simulink model "sim_aut_dual_scen"  (R2025b)
settings: Solver=ode45  StartTime=0.0  StopTime=Tfin  FixedStep=1e-3  MaxStep=1e-2  MinStep=1e-3  RelTol=5e-3
values from neighbouring files (symbols this model uses):
  bp = [-1.25 -1.19897959184 -1.14795918367 -1.09693877551 -1.04591836735 -0.994897959184 -0.94387755102 -0.892857142857 -0.841836734694 -0.790816326531 -0.739795918367 -0.688775510204 ... (50 elements, 1x50)]    [tire_model.mat]
  C1 = 2.7e4    (= 27000)    [main.m]    (also in model.m)
  C2 = 2e4    (= 20000)    [main.m]    (also in model.m)
  Jz = 4000    [main.m]    (also in model.m)
  K = nmpc_design_st2(par,2)    [main.m]
  l1 = 1.2    [main.m]    (also in model.m)
  l2 = 1.6    [main.m]    (also in model.m)
  m = 1575    [main.m]    (also in model.m)
  Np = round(vx_ref*K.Tp/mean(ds))    [main.m]
  pacf = [2550.90487699 2674.70463742 2810.77279096 2960.97362657 3127.55760929 3313.26346728 3521.4532226 3756.29269015 4022.99538347 4328.15571957 4680.20907939 5090.07319782 ... (50 elements, 1x50)]    [tire_model.mat]
  pacr = [2550.90487699 2674.70463742 2810.77279096 2960.97362657 3127.55760929 3313.26346728 3521.4532226 3756.29269015 4022.99538347 4328.15571957 4680.20907939 5090.07319782 ... (50 elements, 1x50)]    [tire_model.mat]
  psi = x(3)    [model.m]
  psir = [atan2(diff(Yr),diff(Xr));0]    [main.m]
  refPoses = [Xr,Yr,psir]    [main.m]
  Ts = 0.05    [main.m]
  ze0 = [X0;Y0;psi0;vx0;vy0;wpsi0]    [main.m]
undefined symbols (not defined in the file or in its folder): aMode, plot_ref, x_o
libraries: autolibsharedcommon x11, autolibshared x5, autolibpowerinfoutils x2, autolibutils x2, sharedtransform x2, simulink x1, drivingscenarioandsensors x1
(part 1 of 4)
settings Model: PacingRate=0.750000  Creator=The MathWorks, Inc.  LastModifiedBy=denni
settings SolverCC: ZeroCrossAlgorithm=Adaptive  AlgebraicLoopSolver=TrustRegion  DecoupledContinuousIntegration=on  MinimalZcImpactIntegration=on
settings DataIOCC: SaveOutput=off  DSMLogging=off  SaveTime=off  ReturnWorkspaceOutputs=off
settings DebuggingCC: UnconnectedInputMsg=warning  UnconnectedOutputMsg=warning  UnconnectedLineMsg=warning  ArithmeticOperatorsInVariantConditions=warning
settings ModelReferenceCC: EnableRefExpFcnMdlSchedulingChecks=on  PropagateSignalLabelsOutOfModel=off
settings SFSimCC: SimUseLocalCustomCode=off  CustomCodeUndefinedFunction=UseInterfaceOnly
settings RTWCC: RTWUseLocalCustomCode=off  GPUComputeCapability=3.5  DLArmComputeVersion=19.05

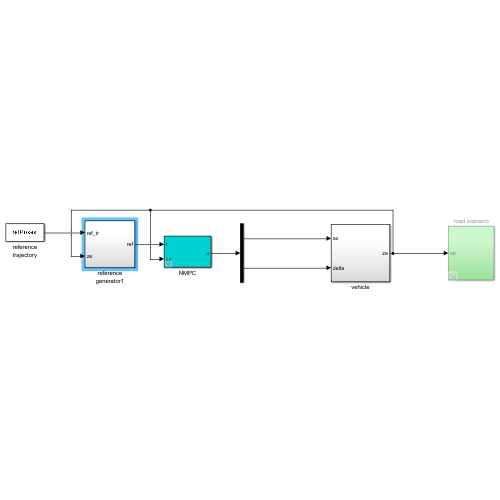
[thumbnail: Simulink's stored preview of the top-level diagram]
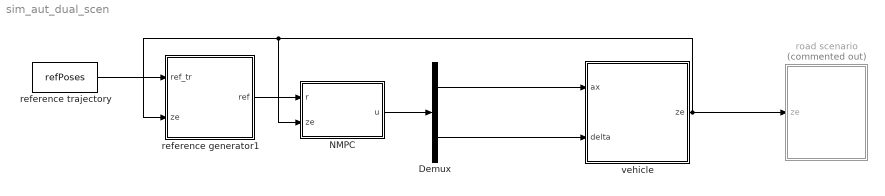
== system sim_aut_dual_scen ==
  Demux : Demux  Outputs=2
  NMPC : Subsystem  mask{K=K}
      mask prompts: K "NMPC structure"
  reference generator1 : Subsystem
  reference trajectory : Constant  Value=refPoses
  road scenario : Subsystem  Commented=on
      settings: PortSchema="{\"entries\":[{\"content\":{\"sides\":[{\"content\":{},\"type\":\"ConnectorPlacement.EquallySpacedRectSide\",\"uuid\":\"f0897155-b1ca-4bdd-a38e-3494662c4a0b\"},{\"content\":{\"connectorIds\":[\"In1\"],\"side\":\"RIGHT\"},\"type\":\"ConnectorPlacement.EquallySpacedRectSide\",\"uuid\":\"ba8f9432-9c07-44a3-8769-5c417be23bfd\"},{\"content\":{\"side\":\"TOP\"},\"type\":\"ConnectorPlacement.EquallySpacedRectSide\",\"uuid\":\"74ba7e9d-4aff-4913-b94c-95c9a4f4fd7f\"}]},\"type\":\"ConnectorPlacement.EquallySpacedConnector\",\"uuid\":\"ef070011-996a-4f52-a3ae-9ceda936acba\"}],\"packageUris\":[\"http://schema.mathworks.com/mf0/Connector/R2020b\"],\"version\":\"1.0\"}"
  vehicle : Subsystem
  wires:
  vehicle/1(ze) -> reference generator1/2(ze), NMPC/2(ze), road scenario/1(ze)
  reference trajectory/1 -> reference generator1/1(ref_tr)
  NMPC/1(u) -> Demux/1
  reference generator1/1(ref) -> NMPC/1(r)
  Demux/2 -> vehicle/2(delta)
  Demux/1 -> vehicle/1(ax)

== system sim_aut_dual_scen/NMPC ==
  r : Inport
  ze : Inport  Port=2
  Clock : Clock
  Mux2 : Mux
  Rate Transition{1..4} (4 alike) : RateTransition  OutPortSampleTime=K.Ts
  Selector1 : Selector  InputPortWidth=K.nc  IndexOptions=Index vector (dialog)  Indices=1:K.nu  OutputSizes=1
  Unit Delay : UnitDelay  InitialCondition=zeros(K.nc,1)  SampleTime=K.Ts  HasFrameUpgradeWarning=on
  nmpc : MATLABFcn  MATLABFcn=nmpc_st2(K,u(1:K.nx),u(K.nx+1:K.nx+K.nc),u(K.nx+K.nc+1:end-1),u(end))  OutputDimensions=K.nc
  u : Outport
  wires:
  ze/1 -> Rate Transition2/1
  Unit Delay/1 -> Mux2/2, Rate Transition1/1
  Mux2/1 -> nmpc/1
  r/1 -> Rate Transition3/1
  Rate Transition2/1 -> Mux2/1
  Rate Transition1/1 -> Selector1/1
  Rate Transition3/1 -> Mux2/3
  nmpc/1 -> Unit Delay/1
  Selector1/1 -> u/1
  Clock/1 -> Rate Transition4/1
  Rate Transition4/1 -> Mux2/4

== system sim_aut_dual_scen/reference generator1 ==
  ref_tr : Inport
  ze : Inport  Port=2
  Constant : Constant  Value=Np
  Demux : Demux
  Gain : Gain  Gain=[0 0 0 3.6 0 0]  Multiplication=Matrix(K*u)
  Gain1 : Gain  Gain=-1
  MATLAB Function1 : MATLAB Function  TreatAsAtomicUnit=on
  Mux : Mux  Inputs=2
  Mux1 : Mux  Inputs=2
  Scope3 : Scope  NumInputPorts=3
      settings: ActiveDisplayYMinimum=-0.12618507931424761  ActiveDisplayYMaximum=0.15446039878025969  DataLoggingVariableName=ScopeData2
  Subsystem : Subsystem
  To Workspace1 : ToWorkspace  VariableName=errors  SaveFormat=Timeseries  SampleTime=-1
  To Workspace2 : ToWorkspace  VariableName=e_ct  SaveFormat=Timeseries  SampleTime=-1
  ref : Outport
  wires:
  ref_tr/1 -> MATLAB Function1/2(ref_tr)
  ze/1 -> Gain/1, Subsystem/3(ze), MATLAB Function1/3(ze)
  MATLAB Function1/2(ref_pose) -> Subsystem/2(ref_pose)
  Subsystem/1(ee) -> Demux/1
  Subsystem/2(e_ct) -> Mux1/1, To Workspace2/1
  Mux/1 -> To Workspace1/1
  Gain/1 -> Scope3/3
  MATLAB Function1/1(ref) -> Subsystem/1(ref XY), ref/1
  Constant/1 -> MATLAB Function1/1(Np)
  Demux/1 -> Gain1/1, Mux/1
  Demux/2 -> Scope3/2, Mux/2
  Mux1/1 -> Scope3/1
  Gain1/1 -> Mux1/2

== system sim_aut_dual_scen/road scenario ==
  ze : Inport
  MATLAB Function1 : MATLAB Function  TreatAsAtomicUnit=on
  Scenario Reader : drivingscenarioandsensors/Scenario Reader  ScenarioSource=From workspace  ScenarioFileName=EgoVehicleGoesStraight.mat  ScenarioVariableName=scenario  OutputCoordinateSystem=Vehicle coordinates  EgoVehicleSource=Input port  EgoVehicleActorID=1  OrientVehiclesOnRoad=on  OutputEgoVehiclePose=on  OutputEgoVehicleState=on  SampleTime=0.1  LaneBoundaryOutput=All lane boundaries  LaneBoundaryDistance=0:0.5:9.5  LaneBoundaryLocation=Center of lane markings  BusNameSource=Auto  BusName=ActorPose  BusNumActorsSource=Scenario  BusNumActors=3  BusName2Source=Auto  BusName2=BusLaneBoundaries  BusNumLaneBoundariesSource=Scenario  BusNumLaneBoundaries=10  BusName3Source=Auto  BusName3=BusEgoActor  BusName4Source=Auto  BusName4=BusEgoState  ShowCoordinateLabels=on  SimulateUsing=Interpreted execution
  Terminator : Terminator
  Terminator1 : Terminator
  wires:
  MATLAB Function1/1(egoPose) -> Scenario Reader/1
  Scenario Reader/1 -> Terminator/1
  Scenario Reader/2 -> Terminator1/1
  ze/1 -> MATLAB Function1/1(ze)

== system sim_aut_dual_scen/vehicle ==
  ax : Inport
  delta : Inport  Port=2
  Actuator : TransferFcn  Denominator=[0.1 1]
  Rate Transition3 : RateTransition  InitialCondition=ze0  OutPortSampleTime=Ts
  Saturation : Saturate  UpperLimit=0.4  LowerLimit=-0.4
  Saturation1 : Saturate  UpperLimit=3  LowerLimit=-10
  Scope1 : Scope  NumInputPorts=2
      settings: ActiveDisplayYMinimum=-11.625  ActiveDisplayYMaximum=4.625
  Scope2 : Scope  NumInputPorts=2
      settings: ActiveDisplayYMinimum=-0.04592  ActiveDisplayYMaximum=0.31381
  To Workspace : ToWorkspace  VariableName=ze  SaveFormat=Timeseries  SampleTime=-1
  To Workspace1 : ToWorkspace  VariableName=delta  SaveFormat=Timeseries  SampleTime=-1
  To Workspace2 : ToWorkspace  VariableName=ax  SaveFormat=Timeseries  SampleTime=-1
  dual-track : Subsystem
  lower level controller/actuators : TransferFcn  Denominator=[0.5 1]
  ze : Outport  VectorParamsAs1DForOutWhenUnconnected=off
  wires:
  Rate Transition3/1 -> To Workspace/1, ze/1
  delta/1 -> To Workspace1/1, Actuator/1
  Actuator/1 -> Saturation/1
  Saturation/1 -> Scope2/2, dual-track/2(delta)
  lower level controller/actuators/1 -> Saturation1/1
  Saturation1/1 -> Scope2/1, dual-track/1(ax), Scope1/2
  ax/1 -> To Workspace2/1, Scope1/1, lower level controller/actuators/1
  dual-track/1(state) -> Rate Transition3/1

== system sim_aut_dual_scen/reference generator1/Subsystem ==
  ref XY : Inport
  ref_pose : Inport  Port=2
  ze : Inport  Port=3
  Discrete Derivative : simulink/Discrete/Discrete Derivative  gainval=1.0  ICPrevScaledInput=psir(1)/Ts  OutMin=[]  OutMax=[]  OutDataType=fixdt(1, 16)  OutScaling=2^-10  DoSatur=off
  Interpreted MATLAB Function : MATLABFcn  Commented=on  MATLABFcn=plot_ref(u)  OutputDimensions=0
  MATLAB Function2 : MATLAB Function  TreatAsAtomicUnit=on  VariantControl=Choice
  Mux : Mux  Inputs=2
  Rate Transition : RateTransition  Commented=on  OutPortSampleTime=Ts
  Selector2 : Selector  InputPortWidth=3  IndexOptions=Index vector (dialog)  Indices=3  OutputSizes=1
  Terminator : Terminator
  errors : Subsystem
  ee : Outport
  e_ct : Outport  Port=2
  wires:
  MATLAB Function2/1(e_ct) -> e_ct/1
  Discrete Derivative/1 -> errors/2(psi_r_dot)
  ze/1 -> MATLAB Function2/2(ze), errors/3(ze), Mux/1
  Rate Transition/1 -> Interpreted MATLAB Function/1
  errors/1(ee) -> ee/1
  ref XY/1 -> Mux/2
  Mux/1 -> Rate Transition/1
  ref_pose/1 -> MATLAB Function2/1(ref_pose), errors/1(refPoses), Selector2/1
  Selector2/1 -> Discrete Derivative/1
  MATLAB Function2/2(e_h) -> Terminator/1

== system sim_aut_dual_scen/vehicle/dual-track ==
  ax : Inport
  delta : Inport  Port=2
  Bus Selector1 : BusSelector  OutputSignals=InertFrm.Cg.Disp.X,InertFrm.Cg.Disp.Y
  Constant1 : Constant  Value=[0;0]
  Gain1 : Gain  Gain=[1;1]
  Gain2 : Gain  Gain=m*[0.5;0.5]
  Mux2 : Mux  Inputs=6
  Terminator1 : Terminator
  Terminator4 : Terminator
  Vehicle Body 3DOF Dual Track : Subsystem  AncestorBlock=autolibshared/Vehicle Body 3DOF Single Track  mask(Vehicle Body 3DOF Lateral){trackMode=Dual, inputMode=External longitudinal forces, frontSteerMode=on, rearSteerMode=off, windMode=off, muMode=off, extFMode=off, extMMode=off, htchFMode=off, htchMMode=off, extXo=off, extpsio=off, extxdoto=off, extro=off, extYo=off, extTamb=off, extydoto=off, aMode=aMode, NF=2, NR=2, m=m, a=l1, b=l2, h=0.35, dh=1, hh=0.2, X_o=ze0(1), xdot_o=ze0(4), CalphaMode=off, sigmaMode=on, d=0, hl=0, w=[1.4,1.4], Cy_f=C1, Cy_r=C2, sigma_f=.1, sigma_r=.1, alpha_f_brk=[-.1 .1], Cy_f_data=[-9e3 9e3], alpha_r_brk=[-.1 .1], Cy_r_data=[-9e3 9e3], Y_o=ze0(2), ydot_o=ze0(5), Izz=Jz, psi_o=ze0(3), r_o=ze0(6), Af=2, Cd=.3, Cl=.1, Cpm=.1, beta_w=[0 0.01:0.01:0.3], Cs=[0 0.01:0.01:0.3], Cym=[0 1e-6:0.01:0.3], Pabs=101325, Tair=273, g=9.81, mu=1, xdot_tol=.01, Fznom=5000, Fxtire_sat=1e6, Fytire_sat=1e6, longOff=0, latOff=0, vertOff=0, wrapAng=off}
      mask prompts: trackMode "autoblks_shared:autoblkVehBody3DofLat:blkPrm_trackMode"; inputMode "autoblks_shared:autoblkVehBody3DofLat:blkPrm_inputMode"; frontSteerMode "autoblks_shared:autoblkVehBody3DofLat:blkPrm_frontSteerMode"; rearSteerMode "autoblks_shared:autoblkVehBody3DofLat:blkPrm_rearSteerMode"; windMode "autoblks_shared:autoblkVehBody3DofLat:blkPrm_windMode"; muMode "autoblks_shared:autoblkVehBody3DofLat:blkPrm_muMode"; extFMode "autoblks_shared:autoblkVehBody3DofLat:blkPrm_extFMode"; extMMode "autoblks_shared:autoblkVehBody3DofLat:blkPrm_extMMode"; htchFMode "autoblks_shared:autoblkVehBody3DofLat:blkPrm_htchFMode"; htchMMode "autoblks_shared:autoblkVehBody3DofLat:blkPrm_htchMMode"; extXo "autoblks_shared:autoblkVehBody3DofLat:blkPrm_extXo"; extpsio "autoblks_shared:autoblkVehBody3DofLat:blkPrm_extpsio"; extxdoto "autoblks_shared:autoblkVehBody3DofLat:blkPrm_extxdoto"; extro "autoblks_shared:autoblkVehBody3DofLat:blkPrm_extro"; extYo "autoblks_shared:autoblkVehBody3DofLat:blkPrm_extYo"; extTamb "autoblks_shared:autoblkVehBody3DofLat:blkPrm_extTamb"; extydoto "autoblks_shared:autoblkVehBody3DofLat:blkPrm_extydoto"; NF "autoblks_shared:autoblkVehBody3DofLat:blkPrm_NF"; NR "autoblks_shared:autoblkVehBody3DofLat:blkPrm_NR"; m "autoblks_shared:autoblkVehBody3DofLat:blkPrm_m"; a "autoblks_shared:autoblkVehBody3DofLat:blkPrm_a"; b "autoblks_shared:autoblkVehBody3DofLat:blkPrm_b"; h "autoblks_shared:autoblkVehBody3DofLat:blkPrm_h"; dh "autoblks_shared:autoblkVehBody3DofLat:blkPrm_dh"; hh "autoblks_shared:autoblkVehBody3DofLat:blkPrm_hh"; X_o "autoblks_shared:autoblkVehBody3DofLat:blkPrm_X_o"; xdot_o "autoblks_shared:autoblkVehBody3DofLat:blkPrm_xdot_o"; CalphaMode "autoblks_shared:autoblkVehBody3DofLat:blkPrm_CalphaMode"; sigmaMode "autoblks_shared:autoblkVehBody3DofLat:blkPrm_sigmaMode"; d "autoblks_shared:autoblkVehBody3DofLat:blkPrm_d"; hl "autoblks_shared:autoblkVehBody3DofLat:blkPrm_hl"; w "autoblks_shared:autoblkVehBody3DofLat:blkPrm_w"; Cy_f "autoblks_shared:autoblkVehBody3DofLat:blkPrm_Cy_f"; Cy_r "autoblks_shared:autoblkVehBody3DofLat:blkPrm_Cy_r"; sigma_f "autoblks_shared:autoblkVehBody3DofLat:blkPrm_sigma_f"; sigma_r "autoblks_shared:autoblkVehBody3DofLat:blkPrm_sigma_r"; alpha_f_brk "autoblks_shared:autoblkVehBody3DofLat:blkPrm_alpha_f_brk"; Cy_f_data "autoblks_shared:autoblkVehBody3DofLat:blkPrm_Cy_f_data"; alpha_r_brk "autoblks_shared:autoblkVehBody3DofLat:blkPrm_alpha_r_brk"; Cy_r_data "autoblks_shared:autoblkVehBody3DofLat:blkPrm_Cy_r_data"; Y_o "autoblks_shared:autoblkVehBody3DofLat:blkPrm_Y_o"; ydot_o "autoblks_shared:autoblkVehBody3DofLat:blkPrm_ydot_o"; Izz "autoblks_shared:autoblkVehBody3DofLat:blkPrm_Izz"; psi_o "autoblks_shared:autoblkVehBody3DofLat:blkPrm_psi_o"; r_o "autoblks_shared:autoblkVehBody3DofLat:blkPrm_r_o"; Af "autoblks_shared:autoblkVehBody3DofLat:blkPrm_Af"; Cd "autoblks_shared:autoblkVehBody3DofLat:blkPrm_Cd"; Cl "autoblks_shared:autoblkVehBody3DofLat:blkPrm_Cl"; Cpm "autoblks_shared:autoblkVehBody3DofLat:blkPrm_Cpm"; beta_w "autoblks_shared:autoblkVehBody3DofLat:blkPrm_beta_w"; Cs "autoblks_shared:autoblkVehBody3DofLat:blkPrm_Cs"; Cym "autoblks_shared:autoblkVehBody3DofLat:blkPrm_Cym"; Pabs "autoblks_shared:autoblkVehBody3DofLat:blkPrm_Pabs"; Tair "autoblks_shared:autoblkVehBody3DofLat:blkPrm_Tair"; g "autoblks_shared:autoblkVehBody3DofLat:blkPrm_g"; mu "autoblks_shared:autoblkVehBody3DofLat:blkPrm_mu"; xdot_tol "autoblks_shared:autoblkVehBody3DofLat:blkPrm_xdot_tol"; Fznom "autoblks_shared:autoblkVehBody3DofLat:blkPrm_Fznom"; Fxtire_sat "autoblks_shared:autoblkVehBody3DofLat:blkPrm_Fxtire_sat"; Fytire_sat "autoblks_shared:autoblkVehBody3DofLat:blkPrm_Fytire_sat"; longOff "autoblks_shared:autoblkVehBody3DofLat:blkPrm_longOff"; latOff "autoblks_shared:autoblkVehBody3DofLat:blkPrm_latOff"; vertOff "autoblks_shared:autoblkVehBody3DofLat:blkPrm_vertOff"; wrapAng "autoblks_shared:autoblkVehBody3DofLat:blkPrm_wrapAng"
      mask help: autoblks_shared:autoblkVehBody3DofLat:blkDesc
      mask init:
      | [~]=autosharedicon('vehdynliblat3dof',gcb,0);
      mask Help: eval('autosharedhelp(''vb3doflat'')');
      mask TypeOptions trackMode: autoblks_shared:autoblkVehBody3DofLat:blkCmb_trackMode_c1 | autoblks_shared:autoblkVehBody3DofLat:blkCmb_trackMode_c2
      mask Callback trackMode: [~]=autosharedicon('vehdynliblat3dof',gcb,5);
      mask TypeOptions inputMode: autoblks_shared:autoblkVehBody3DofLat:blkCmb_inputMode_c1 | autoblks_shared:autoblkVehBody3DofLat:blkCmb_inputMode_c2 | autoblks_shared:autoblkVehBody3DofLat:blkCmb_inputMode_c3
      mask Callback inputMode: [~]=autosharedicon('vehdynliblat3dof',gcb,1);
      mask Callback muMode: [~]=autosharedicon('vehdynliblat3dof',gcb,2);
      mask Callback extXo: [~]=autosharedicon('vehdynliblat3dof',gcb,7);
      mask Callback extpsio: [~]=autosharedicon('vehdynliblat3dof',gcb,7);
      mask Callback extxdoto: [~]=autosharedicon('vehdynliblat3dof',gcb,7);
      mask Callback extro: [~]=autosharedicon('vehdynliblat3dof',gcb,7);
      mask Callback extYo: [~]=autosharedicon('vehdynliblat3dof',gcb,7);
      mask Callback extTamb: [~]=autosharedicon('vehdynliblat3dof',gcb,6);
      mask Callback extydoto: [~]=autosharedicon('vehdynliblat3dof',gcb,7);
      mask Callback CalphaMode: [~]=autosharedicon('vehdynliblat3dof',gcb,3);
      mask Callback sigmaMode: [~]=autosharedicon('vehdynliblat3dof',gcb,4);
      mask DialogControl blockConfig Prompt: autoblks_shared:autoblkVehBody3DofLat:blkDlg_blockConfig
      mask DialogControl trackMode Prompt: Vehicle track:
      mask DialogControl inputMode Prompt: Axle forces:
      mask DialogControl extModePanel Prompt: autoblks_shared:autoblkVehBody3DofLat:blkDlg_extModePanel
      mask DialogControl frontSteerMode Prompt: Front wheel steering
      mask DialogControl rearSteerMode Prompt: Rear wheel steering
      mask DialogControl windMode Prompt: External wind
      mask DialogControl muMode Prompt: External friction
      mask DialogControl extFMode Prompt: External forces
      mask DialogControl extMMode Prompt: External moments
      mask DialogControl htchFMode Prompt: Hitch forces
      mask DialogControl htchMMode Prompt: Hitch moments
      mask DialogControl extXo Prompt: Initial longitudinal position
      mask DialogControl extpsio Prompt: Initial yaw angle
      mask DialogControl extxdoto Prompt: Initial longitudinal velocity
      mask DialogControl extro Prompt: Initial yaw rate
      mask DialogControl extYo Prompt: Initial lateral position
      mask DialogControl extTamb Prompt: Air temperature
      mask DialogControl extydoto Prompt: Initial lateral velocity
      mask DialogControl ParameterGroupVar Prompt: autoblks_shared:autoblkVehBody3DofLat:blkDlg_ParameterGroupVar
      mask DialogControl LongPanel Prompt: autoblks_shared:autoblkVehBody3DofLat:blkDlg_LongPanel
      mask DialogControl NF Prompt: Number of wheels on front axle, NF [-]:
      mask DialogControl NR Prompt: Number of wheels on rear axle, NR [-]:
      mask DialogControl m Prompt: Vehicle mass, m [kg]:
      mask DialogControl a Prompt: Longitudinal distance from center of mass to front axle, a [m]:
      mask DialogControl b Prompt: Longitudinal distance from center of mass to rear axle, b [m]:
      mask DialogControl h Prompt: Vertical distance from center of mass to axle plane, h [m]:
      mask DialogControl dh Prompt: Longitudinal distance from center of mass to hitch, dh [m]:
      mask DialogControl hh Prompt: Vertical distance from hitch to axle plane, hh [m]:
      mask DialogControl X_o Prompt: Initial inertial frame longitudinal position, X_o [m]:
      mask DialogControl xdot_o Prompt: Initial longitudinal velocity, xdot_o [m/s]:
      mask DialogControl LatPanel Prompt: autoblks_shared:autoblkVehBody3DofLat:blkDlg_LatPanel
      mask DialogControl CalphaMode Prompt: Mapped corner stiffness:
      mask DialogControl sigmaMode Prompt: Include relaxation length dynamics:
      mask DialogControl d Prompt: Lateral distance from geometric centerline to center of mass, d [m]:
      mask DialogControl hl Prompt: Lateral distance from geometric centerline to hitch, hl [m]:
      mask DialogControl w Prompt: Track width, w [m]:
      mask DialogControl Cy_f Prompt: Front tire corner stiffness, Cy_f [N/rad]:
      mask DialogControl Cy_r Prompt: Rear tire corner stiffness, Cy_r [N/rad]:
      mask DialogControl sigma_f Prompt: Front tire(s) relaxation length, sigma_f [m]:
      mask DialogControl sigma_r Prompt: Rear tire(s) relaxation length, sigma_r [m]:
      mask DialogControl alpha_f_brk Prompt: Front axle slip angle breakpoints, alpha_f_brk [rad]:
      mask DialogControl Cy_f_data Prompt: Front axle corner data, Cy_f_data [N/rad]:
      mask DialogControl alpha_r_brk Prompt: Rear axle slip angle breakpoints, alpha_r_brk [rad]:
      mask DialogControl Cy_r_data Prompt: Rear axle corner data, Cy_r_data [N/rad]:
      mask DialogControl Y_o Prompt: Initial inertial frame lateral displacement, Y_o [m]:
      mask DialogControl ydot_o Prompt: Initial lateral velocity, ydot_o [m/s]:
      mask DialogControl YawPanel Prompt: autoblks_shared:autoblkVehBody3DofLat:blkDlg_YawPanel
      mask DialogControl Izz Prompt: Yaw polar inertia, Izz [kg*m^2]:
      mask DialogControl psi_o Prompt: Initial yaw angle, psi_o [rad]:
      mask DialogControl r_o Prompt: Initial yaw rate, r_o [rad/s]:
      mask DialogControl AeroParams Prompt: autoblks_shared:autoblkVehBody3DofLat:blkDlg_AeroParams
      mask DialogControl Af Prompt: Longitudinal drag area, Af [m^2]:
      mask DialogControl Cd Prompt: Longitudinal drag coefficient, Cd [-]:
      mask DialogControl Cl Prompt: Longitudinal lift coefficient, Cl [-]:
      mask DialogControl Cpm Prompt: Longitudinal drag pitch moment, Cpm [-]:
      mask DialogControl beta_w Prompt: Relative wind angle vector, beta_w [rad]:
      mask DialogControl Cs Prompt: Side force coefficient vector, Cs [-]:
      mask DialogControl Cym Prompt: Yaw moment coefficient vector, Cym [-]:
      mask DialogControl EnviroPanel Prompt: autoblks_shared:autoblkVehBody3DofLat:blkDlg_EnviroPanel
      mask DialogControl Pabs Prompt: Absolute pressure, Pabs [Pa]:
      mask DialogControl Tair Prompt: Air temperature, Tair [K]:
      mask DialogControl g Prompt: Gravitational acceleration, g [m/s^2]:
      mask DialogControl mu Prompt: Nominal friction scaling factor, mu [-]:
      mask DialogControl SimPanel Prompt: autoblks_shared:autoblkVehBody3DofLat:blkDlg_SimPanel
      mask DialogControl xdot_tol Prompt: Longitudinal velocity tolerance, xdot_tol [m/s]:
      mask DialogControl Fznom Prompt: Nominal normal force, Fznom [N]:
      mask DialogControl Fxtire_sat Prompt: Longitudinal force limit, Fxtire_sat [N]:
      mask DialogControl Fytire_sat Prompt: Lateral force limit, Fytire_sat [N]:
      mask DialogControl longOff Prompt: Geometric longitudinal offset from axle plane, longOff [m]:
      mask DialogControl latOff Prompt: Geometric lateral offset from center plane, latOff [m]:
      mask DialogControl vertOff Prompt: Geometric vertical offset from axle plane, vertOff [m]:
      mask DialogControl wrapAng Prompt: Wrap Euler angles, wrapAng
      mask Display:
      | try
      |     IconInfo = autosharedicon('vehdynliblat3dof',gcb,8);
      | 
      |     image(IconInfo.image, IconInfo.position);
      | 
      |     for i = 1:numel(IconInfo.lconn)
      |         port_label('lconn', i, IconInfo.lconn{i})
      |     end
      | 
      |     for j = 1:numel(IconInfo.rconn)
      |         port_label('rconn', j, IconInfo.rconn{j})
      |     end
      | 
      |     for k = 1:numel(IconInfo.input)
      |         port_label('input', k, IconInfo.input{k})
      |     end
      | 
      |     for m = 1:numel(IconInfo.output)
      |         port_label('output', m, IconInfo.output{m})
      |     end
      | catch
      |     fprintf('Vehicle Body \n 3DOF Lateral')
      | end
  state : Outport
  wires:
  delta/1 -> Gain1/1
  Vehicle Body 3DOF Dual Track/4(psi) -> Mux2/3
  Vehicle Body 3DOF Dual Track/6(FzF) -> Terminator1/1
  Vehicle Body 3DOF Dual Track/5(r) -> Mux2/6
  Vehicle Body 3DOF Dual Track/7(FzR) -> Terminator4/1
  Gain1/1 -> Vehicle Body 3DOF Dual Track/1(WhlAngF)
  Bus Selector1/1 -> Mux2/1  "<X>"
  Vehicle Body 3DOF Dual Track/1(Info) -> Bus Selector1/1
  Constant1/1 -> Vehicle Body 3DOF Dual Track/3(FwR)
  Vehicle Body 3DOF Dual Track/3(ydot) -> Mux2/5
  Vehicle Body 3DOF Dual Track/2(xdot) -> Mux2/4
  ax/1 -> Gain2/1
  Bus Selector1/2 -> Mux2/2  "<Y>"
  Mux2/1 -> state/1  "state"
  Gain2/1 -> Vehicle Body 3DOF Dual Track/2(FwF)

== system sim_aut_dual_scen/reference generator1/Subsystem/errors ==
  refPoses : Inport
  psi_r_dot : Inport  Port=2
  ze : Inport  Port=3
  Integrator : Integrator
  MATLAB Function : MATLAB Function  TreatAsAtomicUnit=on
  Mux : Mux
  ee : Outport
  wires:
  Integrator/1 -> Mux/1
  MATLAB Function/2(e_psi) -> Mux/2
  MATLAB Function/3(e_psi_dot) -> Mux/4
  MATLAB Function/1(e_y_dot) -> Mux/3, Integrator/1
  Mux/1 -> ee/1
  psi_r_dot/1 -> MATLAB Function/2(psi_r_dot)
  ze/1 -> MATLAB Function/3(ze)
  refPoses/1 -> MATLAB Function/1(ref)

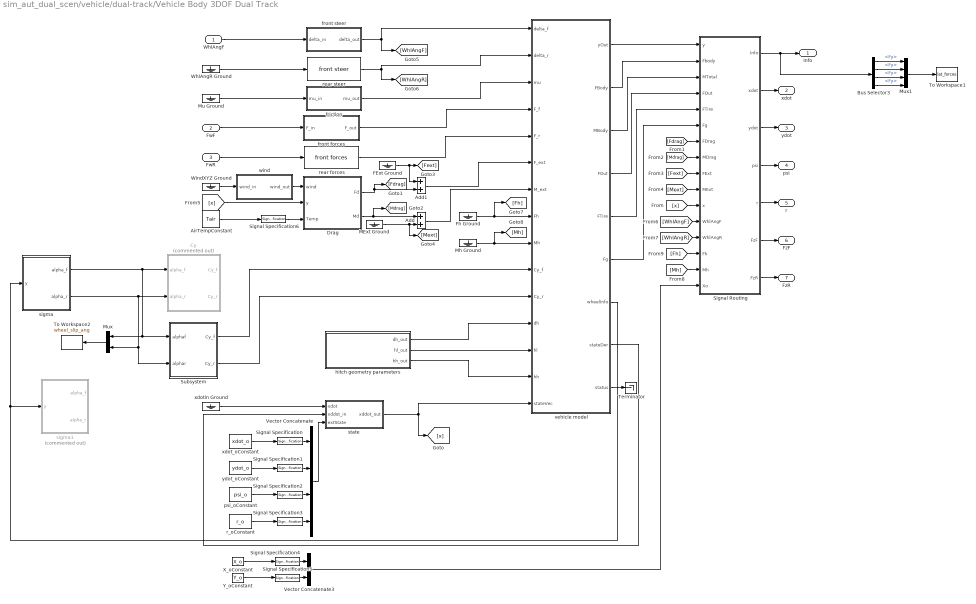
== system sim_aut_dual_scen/vehicle/dual-track/Vehicle Body 3DOF Dual Track ==
  WhlAngF : Inport
  FwF : Inport  Port=2
  FwR : Inport  Port=3
  Add : Sum
  Add1 : Sum
  AirTempConstant : Constant  Value=Tair
  Bus Selector3 : BusSelector  OutputSignals=BdyFrm.Forces.Tires.FrntTires.Lft.Fy,BdyFrm.Forces.Tires.FrntTires.Rght.Fy,BdyFrm.Forces.Tires.RearTires.Lft.Fy,BdyFrm.Forces.Tires.RearTires.Rght.Fy
  Cy : Subsystem  Commented=on  Variant=on  VariantControlMode=label  LabelModeActiveChoice=2
  Drag : Subsystem
  FExt Ground : Ground
  Fh Ground : Ground
  MExt Ground : Ground
  Mh Ground : Ground
  Mu Ground : Ground
  Mux : Mux  Inputs=2
  Mux1 : Mux
  Signal Routing : Subsystem  Variant=on  VariantControlMode=label  LabelModeActiveChoice=1
  Signal Specification : SignalSpecification  Unit=m/s
  Signal Specification1 : SignalSpecification  Unit=m/s
  Signal Specification2 : SignalSpecification  Unit=rad
  Signal Specification3 : SignalSpecification  Unit=rad/s
  Signal Specification4 : SignalSpecification  Unit=m
  Signal Specification5 : SignalSpecification  Unit=m
  Signal Specification6 : SignalSpecification  Unit=K
  Subsystem : Subsystem
  Terminator : Terminator
  To Workspace1 : ToWorkspace  VariableName=lat_forces  SaveFormat=Timeseries  SampleTime=Ts
  To Workspace2 : ToWorkspace  VariableName=wheel_slip_ang  SaveFormat=Timeseries  SampleTime=Ts
  Vector Concatenate : Concatenate  NumInputs=4
  Vector Concatenate3 : Concatenate
  WhlAngR Ground : Ground
  WindXYZ Ground : Ground
  X_oConstant : Constant  Value=X_o
  Y_oConstant : Constant  Value=Y_o
  friction : Subsystem  Variant=on  VariantControlMode=label  LabelModeActiveChoice=2
  front forces : Subsystem  Variant=on  VariantControlMode=label  LabelModeActiveChoice=4
  front steer : Subsystem  Variant=on  VariantControlMode=label  LabelModeActiveChoice=3
  hitch geometry parameters : Subsystem  Variant=on  VariantControlMode=label  LabelModeActiveChoice=3
  psi_oConstant : Constant  Value=psi_o
  r_oConstant : Constant  Value=r_o
  rear forces : autolibshared/Vehicle Body 3DOF Single Track/front forces  SystemSampleTime=-1  LabelModeActiveChoice=4  VariantActivationTime=update diagram  EmptyChoice=off  PassThrough=off  PassThroughVariantControl=(default)  EmptyChoiceVariantControl=(default)  AllowFlexibleInterface=on  Latency=0  AutoFrameSizeCalculation=off
  rear steer : autolibshared/Vehicle Body 3DOF Single Track/front steer  SystemSampleTime=-1  LabelModeActiveChoice=2  VariantActivationTime=update diagram  EmptyChoice=off  PassThrough=off  PassThroughVariantControl=(default)  EmptyChoiceVariantControl=(default)  AllowFlexibleInterface=on  Latency=0  AutoFrameSizeCalculation=off
  sigma : Subsystem  Variant=on  VariantControlMode=label  LabelModeActiveChoice=3
  sigma1 : Subsystem  Commented=on  Variant=on  VariantControlMode=label  LabelModeActiveChoice=3
  state : Subsystem  Variant=on  VariantControlMode=label  LabelModeActiveChoice=0
  vehicle model : MATLAB Function  TreatAsAtomicUnit=on
  wind : Subsystem  Variant=on  VariantControlMode=label  LabelModeActiveChoice=0
  xdot_oConstant : Constant  Value=xdot_o
  xdotin Ground : Ground
  ydot_oConstant : Constant  Value=ydot_o
  Info : Outport  VectorParamsAs1DForOutWhenUnconnected=off
  xdot : Outport  Port=2  VectorParamsAs1DForOutWhenUnconnected=off
  ydot : Outport  Port=3  VectorParamsAs1DForOutWhenUnconnected=off
  psi : Outport  Port=4  VectorParamsAs1DForOutWhenUnconnected=off
  r : Outport  Port=5  VectorParamsAs1DForOutWhenUnconnected=off
  FzF : Outport  Port=6  VectorParamsAs1DForOutWhenUnconnected=off
  FzR : Outport  Port=7  VectorParamsAs1DForOutWhenUnconnected=off
  wires:
  AirTempConstant/1 -> Signal Specification6/1
  [Fh] -> Signal Routing/14(Fh)
  [Mh] -> Signal Routing/15(Mh)
  hitch geometry parameters/3(hh_out) -> vehicle model/14(hh)
  hitch geometry parameters/2(hl_out) -> vehicle model/13(hl)
  hitch geometry parameters/1(dh_out) -> vehicle model/12(dh)
  Mh Ground/1 -> [Mh], vehicle model/9(Mh)
  Fh Ground/1 -> [Fh], vehicle model/8(Fh)
  FExt Ground/1 -> [Fext], Add1/1
  MExt Ground/1 -> Add/2, [Mext]
  FwR/1 -> rear forces/1
  FwF/1 -> front forces/1(F_in)
  xdotin Ground/1 -> state/1(xdot)
  Signal Specification6/1 -> Drag/3(Temp)
  Signal Specification5/1 -> Vector Concatenate3/2
  Y_oConstant/1 -> Signal Specification5/1
  Signal Specification4/1 -> Vector Concatenate3/1
  X_oConstant/1 -> Signal Specification4/1
  Vector Concatenate3/1 -> Signal Routing/16(Xo)
  Signal Specification2/1 -> Vector Concatenate/3
  Signal Specification3/1 -> Vector Concatenate/4
  psi_oConstant/1 -> Signal Specification2/1
  r_oConstant/1 -> Signal Specification3/1
  Signal Specification1/1 -> Vector Concatenate/2
  ydot_oConstant/1 -> Signal Specification1/1
  Signal Specification/1 -> Vector Concatenate/1
  xdot_oConstant/1 -> Signal Specification/1
  Vector Concatenate/1 -> state/3(extState)
  [WhlAngR] -> Signal Routing/13(WhlAngR)
  [WhlAngF] -> Signal Routing/12(WhlAngF)
  Signal Routing/4(psi) -> psi/1
  Mu Ground/1 -> friction/1(mu_in)
  WhlAngR Ground/1 -> rear steer/1
  WhlAngF/1 -> front steer/1(delta_in)
  [x] -> Drag/2(y)
  WindXYZ Ground/1 -> wind/1(wind_in)
  Drag/1(Fd) -> [Fdrag], Add1/2
  wind/1(wind_out) -> Drag/1(wind)
  Drag/2(Md) -> Add/1, [Mdrag]
  rear forces/1 -> vehicle model/5(F_r)
  front forces/1(F_out) -> vehicle model/4(F_f)
  vehicle model/7(wheelInfo) -> sigma/1(y), sigma1/1(y)
  Signal Routing/1(Info) -> Bus Selector3/1, Info/1
  sigma/2(alpha_r) -> Subsystem/2(alphar), Mux/2, Cy/2(alpha_r)
  sigma/1(alpha_f) -> Mux/1, Subsystem/1(alphaf), Cy/1(alpha_f)
  rear steer/1 -> vehicle model/2(delta_r), [WhlAngR]
  front steer/1(delta_out) -> vehicle model/1(delta_f), [WhlAngF]
  friction/1(mu_out) -> vehicle model/3(mu)
  vehicle model/8(stateDer) -> state/2(xddot_in)
  vehicle model/1(yOut) -> Signal Routing/1(y)
  Signal Routing/3(ydot) -> ydot/1
  Signal Routing/5(r) -> r/1
  Signal Routing/6(FzF) -> FzF/1
  Signal Routing/7(FzR) -> FzR/1
  Signal Routing/2(xdot) -> xdot/1
  vehicle model/4(FOut) -> Signal Routing/4(FOut)
  state/1(xddot_out) -> vehicle model/15(stateVec), [x]
  [x] -> Signal Routing/11(x)
  vehicle model/9(status) -> Terminator/1
  vehicle model/5(FTire) -> Signal Routing/5(FTire)
  vehicle model/6(Fg) -> Signal Routing/6(Fg)
  [Fext] -> Signal Routing/9(FExt)
  [Fdrag] -> Signal Routing/7(FDrag)
  [Mdrag] -> Signal Routing/8(MDrag)
  [Mext] -> Signal Routing/10(MExt)
  vehicle model/2(FBody) -> Signal Routing/2(Fbody)
  vehicle model/3(MBody) -> Signal Routing/3(MTotal)
  Add/1 -> vehicle model/7(M_ext)
  Add1/1 -> vehicle model/6(F_ext)
  Subsystem/1(Cy_f) -> vehicle model/10(Cy_f)
  Subsystem/2(Cy_r) -> vehicle model/11(Cy_r)
  Bus Selector3/2 -> Mux1/2  "<Fy>"
  Bus Selector3/3 -> Mux1/3  "<Fy>"
  Bus Selector3/4 -> Mux1/4  "<Fy>"
  Mux1/1 -> To Workspace1/1
  Bus Selector3/1 -> Mux1/1  "<Fy>"
  Mux/1 -> To Workspace2/1

== system sim_aut_dual_scen/vehicle/dual-track/Vehicle Body 3DOF Dual Track/Cy ==
  note: 1) Add Subsystem or Model blocks as valid variant choices.
      | 2) You cannot connect blocks at this level. At simulation, connectivity is automatically
      | determined, based on the active variant and port name matching.
  alpha_f : Inport
  alpha_r : Inport  Port=2
  Cy const : Subsystem  VariantControl=0
  Cy const dual : Subsystem  VariantControl=2
  Cy table : Subsystem  VariantControl=1
  Cy table dual : Subsystem  VariantControl=3
  Cy_f : Outport  VectorParamsAs1DForOutWhenUnconnected=off
  Cy_r : Outport  Port=2  VectorParamsAs1DForOutWhenUnconnected=off

== system sim_aut_dual_scen/vehicle/dual-track/Vehicle Body 3DOF Dual Track/Drag ==
  wind : Inport
  y : Inport  Port=2
  Temp : Inport  Port=3  Unit=K
  Constant : Constant  Value=0
  Demux : Demux  Outputs=3
  Drag Force : autolibsharedcommon/Vehicle Body 3dof/Drag Force  A=Af  beta_w=beta_w  Cd=Cd  Cs=Cs  Cl=Cl  Cpm=Cpm  Lcpm=a+b  Crm=beta_w.*0  Cym=Cym  R=287.058  Pabs=Pabs
  Selector2 : Selector  InputPortWidth=4  IndexOptions=Index vector (dialog)  Indices=[1:3]  OutputSizes=1
  Unary Minus : UnaryMinus
  Unary Minus1 : UnaryMinus
  Vector Concatenate1 : Concatenate  NumInputs=3
  inertial2body : Subsystem
  Fd : Outport  VectorParamsAs1DForOutWhenUnconnected=off
  Md : Outport  Port=2  VectorParamsAs1DForOutWhenUnconnected=off
  wires:
  Temp/1 -> Drag Force/3
  inertial2body/1(Windxyz) -> Drag Force/2
  wind/1 -> inertial2body/2(WindXYZ)
  Demux/3 -> inertial2body/1(psi)
  Demux/1 -> Vector Concatenate1/1
  Demux/2 -> Vector Concatenate1/2
  Constant/1 -> Vector Concatenate1/3
  Vector Concatenate1/1 -> Drag Force/1
  Selector2/1 -> Demux/1
  Drag Force/2 -> Unary Minus1/1
  y/1 -> Selector2/1
  Drag Force/1 -> Unary Minus/1
  Unary Minus/1 -> Fd/1
  Unary Minus1/1 -> Md/1

== system sim_aut_dual_scen/vehicle/dual-track/Vehicle Body 3DOF Dual Track/Signal Routing ==
  note: 1) Add Subsystem or Model blocks as valid variant choices.
      | 2) You cannot connect blocks at this level. At simulation, connectivity is automatically
      | determined, based on the active variant and port name matching.
  y : Inport
  Fbody : Inport  Port=2  Unit=N
  MTotal : Inport  Port=3  Unit=N*m
  FOut : Inport  Port=4
  FTire : Inport  Port=5  Unit=N
  Fg : Inport  Port=6  Unit=N
  FDrag : Inport  Port=7  Unit=N
  MDrag : Inport  Port=8  Unit=N*m
  FExt : Inport  Port=9  Unit=N
  MExt : Inport  Port=10  Unit=N*m
  x : Inport  Port=11
  WhlAngF : Inport  Port=12
  WhlAngR : Inport  Port=13
  Fh : Inport  Port=14  Unit=N
  Mh : Inport  Port=15  Unit=N*m
  Xo : Inport  Port=16
  Signal Routing : Subsystem  VariantControl=0
  Signal Routing Dual : Subsystem  VariantControl=1
  Info : Outport  VectorParamsAs1DForOutWhenUnconnected=off
  xdot : Outport  Port=2  VectorParamsAs1DForOutWhenUnconnected=off
  ydot : Outport  Port=3  VectorParamsAs1DForOutWhenUnconnected=off
  psi : Outport  Port=4  VectorParamsAs1DForOutWhenUnconnected=off
  r : Outport  Port=5  VectorParamsAs1DForOutWhenUnconnected=off
  FzF : Outport  Port=6  VectorParamsAs1DForOutWhenUnconnected=off
  FzR : Outport  Port=7  VectorParamsAs1DForOutWhenUnconnected=off

== system sim_aut_dual_scen/vehicle/dual-track/Vehicle Body 3DOF Dual Track/Subsystem ==
  alphaf : Inport
  alphar : Inport  Port=2
  Cy_f(alpha_f) : Lookup_n-D  NumberOfTableDimensions=1  BreakpointsForDimension1=bp  Table=pacf  ExtrapMethod=Clip  InternalRulePriority=Speed  RndMeth=Simplest
  Cy_r(alpha_r) : Lookup_n-D  NumberOfTableDimensions=1  BreakpointsForDimension1=bp  Table=pacr  ExtrapMethod=Clip  InternalRulePriority=Speed  RndMeth=Simplest
  Cyf : Constant  Commented=on  Value=[Cy_f;Cy_f]
  Cyf1 : Constant  Commented=on  Value=[Cy_r;Cy_r]
  Cy_f : Outport
  Cy_r : Outport  Port=2
  wires:
  alphaf/1 -> Cy_f(alpha_f)/1
  alphar/1 -> Cy_r(alpha_r)/1
  Cy_r(alpha_r)/1 -> Cy_r/1
  Cy_f(alpha_f)/1 -> Cy_f/1

== system sim_aut_dual_scen/vehicle/dual-track/Vehicle Body 3DOF Dual Track/friction ==
  note: 1) Add Subsystem or Model blocks as valid variant choices.
      | 2) You cannot connect blocks at this level. At simulation, connectivity is automatically
      | determined, based on the active variant and port name matching.
  mu_in : Inport  Unit=1
  mu ext : Subsystem  VariantControl=1
  mu ext dual : Subsystem  VariantControl=3
  mu int : Subsystem  VariantControl=0
  mu int dual : Subsystem  VariantControl=2
  mu_out : Outport  Unit=1  VectorParamsAs1DForOutWhenUnconnected=off

== system sim_aut_dual_scen/vehicle/dual-track/Vehicle Body 3DOF Dual Track/front forces ==
  note: 1) Add Subsystem or Model blocks as valid variant choices.
      | 2) You cannot connect blocks at this level. At simulation, connectivity is automatically
      | determined, based on the active variant and port name matching.
  F_in : Inport  Unit=N
  ext : Subsystem  VariantControl=2
  ext dual : Subsystem  VariantControl=5
  ext long : Subsystem  VariantControl=1
  ext long dual : Subsystem  VariantControl=4
  int : Subsystem  VariantControl=0
  int dual : Subsystem  VariantControl=3
  F_out : Outport  Unit=N  VectorParamsAs1DForOutWhenUnconnected=off

== system sim_aut_dual_scen/vehicle/dual-track/Vehicle Body 3DOF Dual Track/front steer ==
  note: 1) Add Subsystem or Model blocks as valid variant choices.
      | 2) You cannot connect blocks at this level. At simulation, connectivity is automatically
      | determined, based on the active variant and port name matching.
  delta_in : Inport  Unit=rad
  delta ext : Subsystem  VariantControl=1
  delta ext dual : Subsystem  VariantControl=3
  delta int : Subsystem  VariantControl=0
  delta int dual : Subsystem  VariantControl=2
  delta_out : Outport  Unit=rad  VectorParamsAs1DForOutWhenUnconnected=off

== system sim_aut_dual_scen/vehicle/dual-track/Vehicle Body 3DOF Dual Track/hitch geometry parameters ==
  note: 1) Add Subsystem or Model blocks as valid variant choices.
      | 2) You cannot connect blocks at this level. At simulation, connectivity is automatically
      | determined, based on the active variant and port name matching.
  hitch active bicycle : Subsystem  VariantControl=1
  hitch active dual track : Subsystem  VariantControl=2
  hitch inactive : Subsystem  VariantControl=3
  dh_out : Outport  Unit=m  VectorParamsAs1DForOutWhenUnconnected=off
  hl_out : Outport  Port=2  Unit=m  VectorParamsAs1DForOutWhenUnconnected=off
  hh_out : Outport  Port=3  Unit=m  VectorParamsAs1DForOutWhenUnconnected=off

== system sim_aut_dual_scen/vehicle/dual-track/Vehicle Body 3DOF Dual Track/sigma ==
  note: 1) Add Subsystem or Model blocks as valid variant choices.
      | 2) You cannot connect blocks at this level. At simulation, connectivity is automatically
      | determined, based on the active variant and port name matching.
  y : Inport
  no sigma : Subsystem  VariantControl=0
  no sigma dual : Subsystem  VariantControl=2
  sigma : Subsystem  VariantControl=1
  sigma dual : Subsystem  VariantControl=3
  alpha_f : Outport  VectorParamsAs1DForOutWhenUnconnected=off
  alpha_r : Outport  Port=2  VectorParamsAs1DForOutWhenUnconnected=off

== system sim_aut_dual_scen/vehicle/dual-track/Vehicle Body 3DOF Dual Track/sigma1 ==
  note: 1) Add Subsystem or Model blocks as valid variant choices.
      | 2) You cannot connect blocks at this level. At simulation, connectivity is automatically
      | determined, based on the active variant and port name matching.
  y : Inport
  no sigma : Subsystem  VariantControl=0
  no sigma dual : Subsystem  VariantControl=2
  sigma : Subsystem  VariantControl=1
  sigma dual : Subsystem  VariantControl=3
  alpha_f : Outport  VectorParamsAs1DForOutWhenUnconnected=off
  alpha_r : Outport  Port=2  VectorParamsAs1DForOutWhenUnconnected=off

== system sim_aut_dual_scen/vehicle/dual-track/Vehicle Body 3DOF Dual Track/state ==
  note: 1) Add Subsystem or Model blocks as valid variant choices.
      | 2) You cannot connect blocks at this level. At simulation, connectivity is automatically
      | determined, based on the active variant and port name matching.
  xdot : Inport  Unit=m/s
  xddot_in : Inport  Port=2  PortDimensions=4
  extState : Inport  Port=3
  xdot ext : Subsystem  VariantControl=1
  xdot int : Subsystem  VariantControl=0
  xddot_out : Outport  VectorParamsAs1DForOutWhenUnconnected=off

== system sim_aut_dual_scen/vehicle/dual-track/Vehicle Body 3DOF Dual Track/wind ==
  note: 1) Add Subsystem or Model blocks as valid variant choices.
      | 2) You cannot connect blocks at this level. At simulation, connectivity is automatically
      | determined, based on the active variant and port name matching.
  wind_in : Inport  Unit=m/s
  wind ext : Subsystem  VariantControl=1
  wind int : Subsystem  VariantControl=0
  wind_out : Outport  Unit=m/s  VectorParamsAs1DForOutWhenUnconnected=off

== system sim_aut_dual_scen/vehicle/dual-track/Vehicle Body 3DOF Dual Track/Cy/Cy const ==
  Cyf : Constant  Value=Cy_f
  Cyr : Constant  Value=Cy_r
  Cy_f : Outport  VectorParamsAs1DForOutWhenUnconnected=off
  Cy_r : Outport  Port=2  VectorParamsAs1DForOutWhenUnconnected=off
  wires:
  Cyr/1 -> Cy_r/1
  Cyf/1 -> Cy_f/1

== system sim_aut_dual_scen/vehicle/dual-track/Vehicle Body 3DOF Dual Track/Cy/Cy const dual ==
  Cyf : Constant  Value=Cy_f
  Cyr : Constant  Value=Cy_r
  Vector Concatenate1 : Concatenate
  Vector Concatenate2 : Concatenate  ConcatenateDimension=2
  Cy_f : Outport  VectorParamsAs1DForOutWhenUnconnected=off
  Cy_r : Outport  Port=2  VectorParamsAs1DForOutWhenUnconnected=off
  wires:
  Cyf/1 -> Vector Concatenate2/2, Vector Concatenate2/1
  Cyr/1 -> Vector Concatenate1/2, Vector Concatenate1/1
  Vector Concatenate2/1 -> Cy_f/1
  Vector Concatenate1/1 -> Cy_r/1

== system sim_aut_dual_scen/vehicle/dual-track/Vehicle Body 3DOF Dual Track/Cy/Cy table ==
  alpha_f : Inport
  alpha_r : Inport  Port=2
  Cy_f(alpha_f) : Lookup_n-D  NumberOfTableDimensions=1  BreakpointsForDimension1=alpha_f_brk  Table=Cy_f_data  ExtrapMethod=Clip  InternalRulePriority=Speed  RndMeth=Simplest
  Cy_r(alpha_r) : Lookup_n-D  NumberOfTableDimensions=1  BreakpointsForDimension1=alpha_r_brk  Table=Cy_r_data  ExtrapMethod=Clip  InternalRulePriority=Speed  RndMeth=Simplest
  Cy_f : Outport  VectorParamsAs1DForOutWhenUnconnected=off
  Cy_r : Outport  Port=2  VectorParamsAs1DForOutWhenUnconnected=off
  wires:
  alpha_r/1 -> Cy_r(alpha_r)/1
  alpha_f/1 -> Cy_f(alpha_f)/1
  Cy_r(alpha_r)/1 -> Cy_r/1
  Cy_f(alpha_f)/1 -> Cy_f/1

== system sim_aut_dual_scen/vehicle/dual-track/Vehicle Body 3DOF Dual Track/Cy/Cy table dual ==
  alpha_f : Inport
  alpha_r : Inport  Port=2
  For Each Subsystem : Subsystem  TreatAsAtomicUnit=on
  Cy_f : Outport  VectorParamsAs1DForOutWhenUnconnected=off
  Cy_r : Outport  Port=2  VectorParamsAs1DForOutWhenUnconnected=off
  wires:
  alpha_r/1 -> For Each Subsystem/2(alpha_r)
  alpha_f/1 -> For Each Subsystem/1(alpha_f)
  For Each Subsystem/2(Cy_r) -> Cy_r/1
  For Each Subsystem/1(Cy_f) -> Cy_f/1

== system sim_aut_dual_scen/vehicle/dual-track/Vehicle Body 3DOF Dual Track/Drag/inertial2body ==
  psi : Inport
  WindXYZ : Inport  Port=2
  Add : Sum
  Add1 : Sum  Inputs=-+
  Demux1 : Demux  Outputs=3
  Product{,1..3} (4 alike) : Product
  Trigonometric Function : Trigonometry  Operator=sincos
  Vector Concatenate2 : Concatenate  NumInputs=3
  Windxyz : Outport  VectorParamsAs1DForOutWhenUnconnected=off
  wires:
  psi/1 -> Trigonometric Function/1
  WindXYZ/1 -> Demux1/1
  Product1/1 -> Add/2
  Demux1/3 -> Vector Concatenate2/3
  Product3/1 -> Add/1
  Add/1 -> Vector Concatenate2/1
  Add1/1 -> Vector Concatenate2/2
  Vector Concatenate2/1 -> Windxyz/1
  Product/1 -> Add1/1
  Product2/1 -> Add1/2
  Trigonometric Function/1 -> Product/1, Product1/1
  Trigonometric Function/2 -> Product2/1, Product3/1
  Demux1/1 -> Product/2, Product3/2
  Demux1/2 -> Product1/2, Product2/2

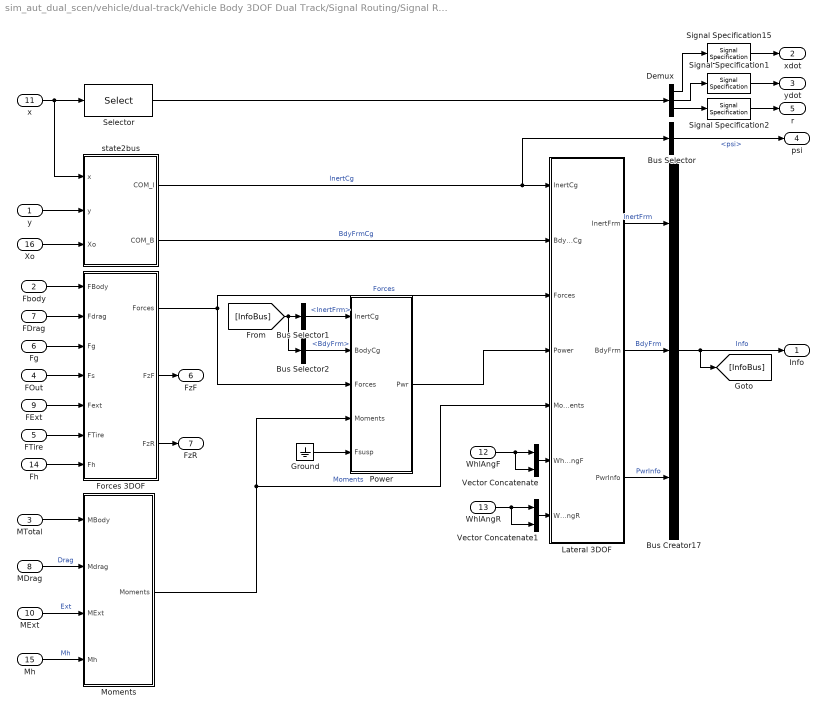
== system sim_aut_dual_scen/vehicle/dual-track/Vehicle Body 3DOF Dual Track/Signal Routing/Signal Routing ==
  y : Inport  PortDimensions=3
  Fbody : Inport  Port=2
  MTotal : Inport  Port=3
  FOut : Inport  Port=4  PortDimensions=6
  FTire : Inport  Port=5
  Fg : Inport  Port=6
  FDrag : Inport  Port=7
  MDrag : Inport  Port=8
  FExt : Inport  Port=9
  MExt : Inport  Port=10
  x : Inport  Port=11
  WhlAngF : Inport  Port=12
  WhlAngR : Inport  Port=13
  Fh : Inport  Port=14
  Mh : Inport  Port=15
  Xo : Inport  Port=16
  Bus Creator17 : BusCreator  Inputs=3
  Bus Selector : BusSelector  OutputSignals=Ang.psi
  Bus Selector1 : BusSelector  OutputSignals=InertFrm
  Bus Selector2 : BusSelector  OutputSignals=BdyFrm
  Demux : Demux  Outputs=3
  Forces 3DOF : Subsystem  VariantControl=2
  Ground : Ground
  Lateral 3DOF : Subsystem  VariantControl=3  mask(Longitudinal 3DOF){aMode=aMode}
  Moments : Subsystem
  Power : Subsystem  VariantControl=3
  Selector : Selector  IndexOptions=Index vector (dialog)  Indices=[1,2,4]  OutputSizes=1
  Signal Specification1 : SignalSpecification  Unit=m/s
  Signal Specification15 : SignalSpecification  Unit=m/s
  Signal Specification2 : SignalSpecification  Unit=rad/s
  Vector Concatenate : Concatenate
  Vector Concatenate1 : Concatenate
  state2bus : Subsystem
  Info : Outport  VectorParamsAs1DForOutWhenUnconnected=off
  xdot : Outport  Port=2  VectorParamsAs1DForOutWhenUnconnected=off
  ydot : Outport  Port=3  VectorParamsAs1DForOutWhenUnconnected=off
  psi : Outport  Port=4  VectorParamsAs1DForOutWhenUnconnected=off
  r : Outport  Port=5  VectorParamsAs1DForOutWhenUnconnected=off
  FzF : Outport  Port=6  VectorParamsAs1DForOutWhenUnconnected=off
  FzR : Outport  Port=7  VectorParamsAs1DForOutWhenUnconnected=off
  wires:
  Fh/1 -> Forces 3DOF/7(Fh)
  FDrag/1 -> Forces 3DOF/2(Fdrag)
  Mh/1 -> Moments/4(Mh)  "Mh"
  Bus Selector/1 -> psi/1  "<psi>"
  Ground/1 -> Power/5(Fsusp)
  Bus Selector2/1 -> Power/2(BodyCg)  "<BdyFrm>"
  Bus Selector1/1 -> Power/1(InertCg)  "<InertFrm>"
  [InfoBus] -> Bus Selector2/1, Bus Selector1/1
  Lateral 3DOF/3(PwrInfo) -> Bus Creator17/3  "PwrInfo"
  Xo/1 -> state2bus/3(Xo)
  Vector Concatenate1/1 -> Lateral 3DOF/7(WhlAngR)
  Vector Concatenate/1 -> Lateral 3DOF/6(WhlAngF)
  WhlAngF/1 -> Vector Concatenate/1, Vector Concatenate/2
  WhlAngR/1 -> Vector Concatenate1/1, Vector Concatenate1/2
  state2bus/2(COM_B) -> Lateral 3DOF/2(BdyFrmCg)  "BdyFrmCg"
  state2bus/1(COM_I) -> Lateral 3DOF/1(InertCg), Bus Selector/1  "InertCg"
  Lateral 3DOF/1(InertFrm) -> Bus Creator17/1  "InertFrm"
  Bus Creator17/1 -> Info/1, [InfoBus]  "Info"
  y/1 -> state2bus/2(y)
  Selector/1 -> Demux/1
  Demux/1 -> Signal Specification15/1
  Demux/2 -> Signal Specification1/1
  Demux/3 -> Signal Specification2/1
  x/1 -> Selector/1, state2bus/1(x)
  Signal Specification15/1 -> xdot/1
  Signal Specification1/1 -> ydot/1
  Signal Specification2/1 -> r/1
  Lateral 3DOF/2(BdyFrm) -> Bus Creator17/2  "BdyFrm"
  Fg/1 -> Forces 3DOF/3(Fg)
  FTire/1 -> Forces 3DOF/6(FTire)
  Forces 3DOF/1(Forces) -> Lateral 3DOF/3(Forces), Power/3(Forces)  "Forces"
  FOut/1 -> Forces 3DOF/4(Fs)
  Forces 3DOF/2(FzF) -> FzF/1
  Forces 3DOF/3(FzR) -> FzR/1
  FExt/1 -> Forces 3DOF/5(Fext)
  Moments/1(Moments) -> Lateral 3DOF/5(Moments), Power/4(Moments)  "Moments"
  MExt/1 -> Moments/3(MExt)  "Ext"
  Power/1(Pwr) -> Lateral 3DOF/4(Power)
  Fbody/1 -> Forces 3DOF/1(FBody)
  MDrag/1 -> Moments/2(Mdrag)  "Drag"
  MTotal/1 -> Moments/1(MBody)

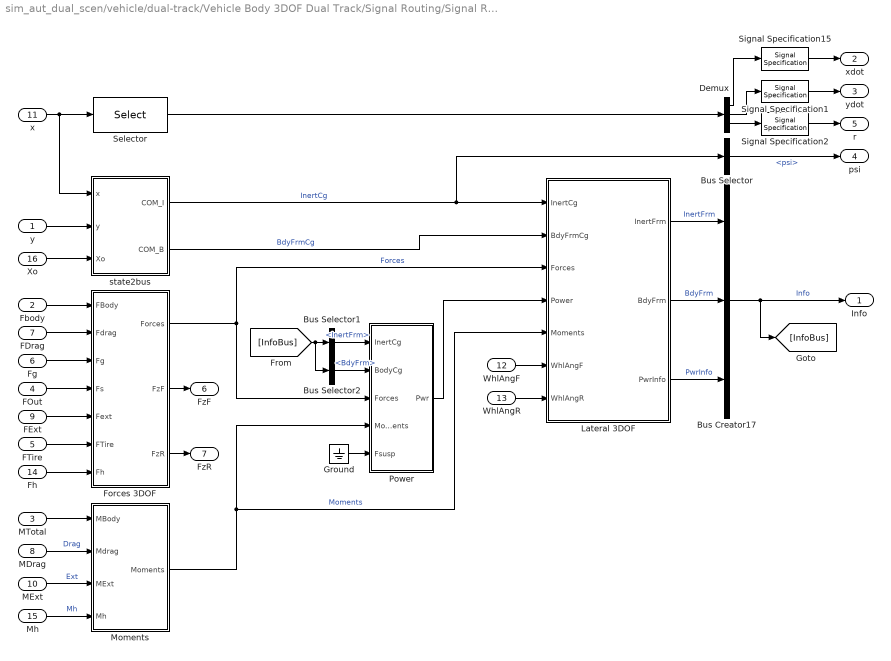
== system sim_aut_dual_scen/vehicle/dual-track/Vehicle Body 3DOF Dual Track/Signal Routing/Signal Routing Dual ==
  y : Inport
  Fbody : Inport  Port=2
  MTotal : Inport  Port=3
  FOut : Inport  Port=4
  FTire : Inport  Port=5
  Fg : Inport  Port=6
  FDrag : Inport  Port=7
  MDrag : Inport  Port=8
  FExt : Inport  Port=9
  MExt : Inport  Port=10
  x : Inport  Port=11
  WhlAngF : Inport  Port=12
  WhlAngR : Inport  Port=13
  Fh : Inport  Port=14
  Mh : Inport  Port=15
  Xo : Inport  Port=16
  Bus Creator17 : BusCreator  Inputs=3
  Bus Selector : BusSelector  OutputSignals=Ang.psi
  Bus Selector1 : BusSelector  OutputSignals=InertFrm
  Bus Selector2 : BusSelector  OutputSignals=BdyFrm
  Demux : Demux  Outputs=3
  Forces 3DOF : Subsystem  VariantControl=2
  Ground : Ground
  Lateral 3DOF : Subsystem  VariantControl=2
  Moments : Subsystem
  Power : Subsystem  VariantControl=4
  Selector : Selector  IndexOptions=Index vector (dialog)  Indices=[1,2,4]  OutputSizes=1
  Signal Specification1 : SignalSpecification  Unit=m/s
  Signal Specification15 : SignalSpecification  Unit=m/s
  Signal Specification2 : SignalSpecification  Unit=rad/s
  state2bus : Subsystem
  Info : Outport  VectorParamsAs1DForOutWhenUnconnected=off
  xdot : Outport  Port=2  VectorParamsAs1DForOutWhenUnconnected=off
  ydot : Outport  Port=3  VectorParamsAs1DForOutWhenUnconnected=off
  psi : Outport  Port=4  VectorParamsAs1DForOutWhenUnconnected=off
  r : Outport  Port=5  VectorParamsAs1DForOutWhenUnconnected=off
  FzF : Outport  Port=6  VectorParamsAs1DForOutWhenUnconnected=off
  FzR : Outport  Port=7  VectorParamsAs1DForOutWhenUnconnected=off
  wires:
  Fh/1 -> Forces 3DOF/7(Fh)
  FTire/1 -> Forces 3DOF/6(FTire)
  Mh/1 -> Moments/4(Mh)  "Mh"
  Bus Selector/1 -> psi/1  "<psi>"
  Demux/3 -> Signal Specification2/1
  Ground/1 -> Power/5(Fsusp)
  Lateral 3DOF/3(PwrInfo) -> Bus Creator17/3  "PwrInfo"
  Bus Selector1/1 -> Power/1(InertCg)  "<InertFrm>"
  [InfoBus] -> Bus Selector2/1, Bus Selector1/1
  Bus Selector2/1 -> Power/2(BodyCg)  "<BdyFrm>"
  Xo/1 -> state2bus/3(Xo)
  WhlAngR/1 -> Lateral 3DOF/7(WhlAngR)
  WhlAngF/1 -> Lateral 3DOF/6(WhlAngF)
  MTotal/1 -> Moments/1(MBody)
  MDrag/1 -> Moments/2(Mdrag)  "Drag"
  Fbody/1 -> Forces 3DOF/1(FBody)
  Power/1(Pwr) -> Lateral 3DOF/4(Power)
  MExt/1 -> Moments/3(MExt)  "Ext"
  Moments/1(Moments) -> Lateral 3DOF/5(Moments), Power/4(Moments)  "Moments"
  FExt/1 -> Forces 3DOF/5(Fext)
  Forces 3DOF/3(FzR) -> FzR/1
  Forces 3DOF/2(FzF) -> FzF/1
  FDrag/1 -> Forces 3DOF/2(Fdrag)
  FOut/1 -> Forces 3DOF/4(Fs)
  Forces 3DOF/1(Forces) -> Lateral 3DOF/3(Forces), Power/3(Forces)  "Forces"
  Fg/1 -> Forces 3DOF/3(Fg)
  Lateral 3DOF/2(BdyFrm) -> Bus Creator17/2  "BdyFrm"
  Signal Specification2/1 -> r/1
  Signal Specification1/1 -> ydot/1
  Signal Specification15/1 -> xdot/1
  x/1 -> Selector/1, state2bus/1(x)
  state2bus/2(COM_B) -> Lateral 3DOF/2(BdyFrmCg)  "BdyFrmCg"
  state2bus/1(COM_I) -> Bus Selector/1, Lateral 3DOF/1(InertCg)  "InertCg"
  Demux/2 -> Signal Specification1/1
  Demux/1 -> Signal Specification15/1
  Selector/1 -> Demux/1
  y/1 -> state2bus/2(y)
  Bus Creator17/1 -> Info/1, [InfoBus]  "Info"
  Lateral 3DOF/1(InertFrm) -> Bus Creator17/1  "InertFrm"

== system sim_aut_dual_scen/vehicle/dual-track/Vehicle Body 3DOF Dual Track/friction/mu ext ==
  mu_in : Inport  Unit=1
  Signal Specification1 : SignalSpecification  Unit=1
  Unit Conversion2 : UnitConversion
  mu_out : Outport  Unit=1  VectorParamsAs1DForOutWhenUnconnected=off
  wires:
  Signal Specification1/1 -> mu_out/1
  mu_in/1 -> Unit Conversion2/1
  Unit Conversion2/1 -> Signal Specification1/1
